simulink model "Control_Seguimiento_de_linea"  (R2023b)
settings: Solver=VariableStepAuto  StartTime=0.0  StopTime=90  RelTol=1e-3
settings Model: Creator=daroc  LastModifiedBy=daroc

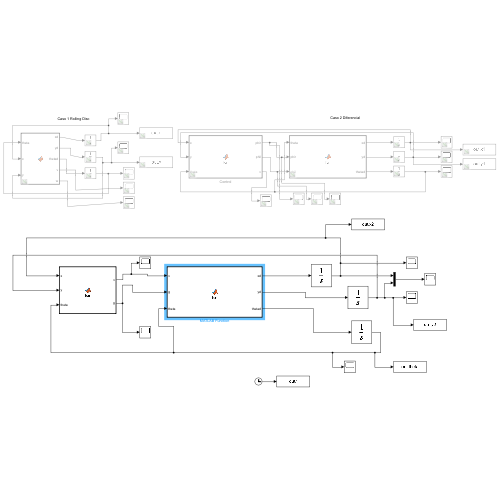
[thumbnail: Simulink's stored preview of the top-level diagram]
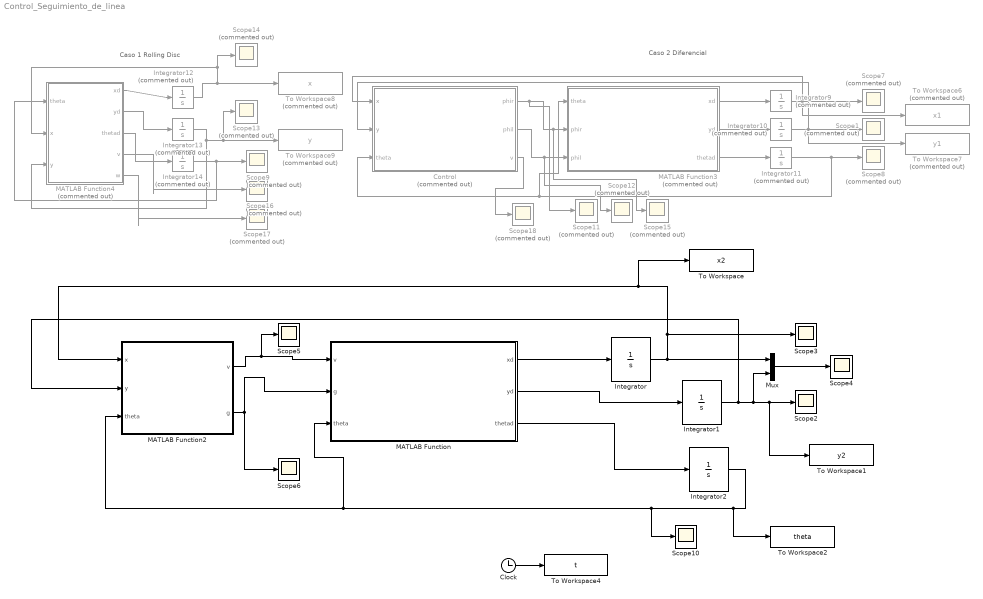
== system Control_Seguimiento_de_linea ==
  note: Caso 1 Rolling Disc
  note: Caso 2 Diferencial
  Clock : Clock
  Control : MATLAB Function  Commented=on  TreatAsAtomicUnit=on
  Integrator : Integrator  InitialCondition=2
  Integrator1 : Integrator  InitialCondition=2
  Integrator{9..14} (6 alike) : Integrator  Commented=on
  Integrator2 : Integrator  InitialCondition=pi/4
  MATLAB Function : MATLAB Function  TreatAsAtomicUnit=on
  MATLAB Function2 : MATLAB Function  TreatAsAtomicUnit=on
  MATLAB Function3 : MATLAB Function  Commented=on  TreatAsAtomicUnit=on
  MATLAB Function4 : MATLAB Function  Commented=on  TreatAsAtomicUnit=on
  Mux : Mux  Inputs=2
  Scope{1,7..9,11..18} (12 alike) : Scope  Commented=on
  Scope{2..6,10} (6 alike) : Scope
  To Workspace : ToWorkspace  VariableName=x2  SampleTime=-1
  To Workspace1 : ToWorkspace  VariableName=y2  SampleTime=-1
  To Workspace2 : ToWorkspace  VariableName=theta  SampleTime=-1
  To Workspace4 : ToWorkspace  VariableName=t  SampleTime=-1
  To Workspace6 : ToWorkspace  Commented=on  VariableName=x1  SampleTime=-1
  To Workspace7 : ToWorkspace  Commented=on  VariableName=y1  SampleTime=-1
  To Workspace8 : ToWorkspace  Commented=on  VariableName=x  SampleTime=-1
  To Workspace9 : ToWorkspace  Commented=on  VariableName=y  SampleTime=-1
  wires:
  MATLAB Function4/1(xd) -> Integrator12/1
  Integrator13/1 -> MATLAB Function4/3(y), Scope13/1, To Workspace9/1
  MATLAB Function4/2(yd) -> Integrator13/1
  Integrator14/1 -> Scope9/1, MATLAB Function4/1(theta)
  Integrator12/1 -> MATLAB Function4/2(x), Scope14/1, To Workspace8/1
  MATLAB Function4/3(thetad) -> Integrator14/1
  Integrator10/1 -> Scope1/1, To Workspace7/1, Control/2(y)
  MATLAB Function3/3(thetad) -> Integrator11/1
  MATLAB Function3/1(xd) -> Integrator9/1
  Integrator11/1 -> MATLAB Function3/1(theta), Control/3(theta), Scope8/1
  Integrator9/1 -> Control/1(x), To Workspace6/1, Scope7/1
  MATLAB Function3/2(yd) -> Integrator10/1
  Control/2(phil) -> Scope12/1, MATLAB Function3/3(phil)
  Control/1(phir) -> Scope11/1, Scope15/1, MATLAB Function3/2(phir)
  MATLAB Function2/1(v) -> MATLAB Function/1(v), Scope5/1
  Integrator2/1 -> To Workspace2/1, Scope10/1, MATLAB Function2/3(theta), MATLAB Function/3(theta)
  Integrator1/1 -> MATLAB Function2/2(y), Mux/2, To Workspace1/1, Scope2/1
  Integrator/1 -> Scope3/1, MATLAB Function2/1(x), To Workspace/1, Mux/1
  MATLAB Function/1(xd) -> Integrator/1
  MATLAB Function/3(thetad) -> Integrator2/1
  MATLAB Function2/2(g) -> Scope6/1, MATLAB Function/2(g)
  Clock/1 -> To Workspace4/1
  Mux/1 -> Scope4/1
  MATLAB Function/2(yd) -> Integrator1/1
  MATLAB Function4/4(v) -> Scope16/1
  MATLAB Function4/5(w) -> Scope17/1
  Control/3(v) -> Scope18/1

== matlab function Control_Seguimiento_de_linea/MATLAB Function ==
  data: v input; xd output; yd output; thetad output; g input; theta input
function [xd,yd,thetad] = fcn(v,g,theta)

L = 0.5;
Rb = L/tan(g);

xd=v*cos(theta);
yd=v*sin(theta);
thetad=v/Rb;

== matlab function Control_Seguimiento_de_linea/Control ==
  data: phir output; phil output; x input; y input; theta input; v output
function [phir,phil,v] = fcn(x,y,theta)

a = 1/5;
b = 1;
c = 1/5;
Kd = 0.7;
Kh = 0.7;
l = 0.5;
r = 0.1;
v = 0.5;

d = ([a b c])*[x; y; 1]/sqrt(a^2+b^2);
alpha_d = -Kd*d;
theta_des = atan2(-a,b);
deltaTheta = theta_des - theta;
alpha_h = Kh*deltaTheta;
w = alpha_d+alpha_h;
phir = (v/r)+(w/r)*(l/2);
phil = (v/r)-(w/r)*(l/2);

== matlab function Control_Seguimiento_de_linea/MATLAB Function2 ==
  data: x input; v output; y input; g output; theta input
function [v, g] = fcn(x,y,theta)

a = 1;
b = 1;
c = -8;
Kd = 0.7;
Kh = 0.7;

v = 0.5;

d = ([a b c])*[x; y; 1]/sqrt(a^2+b^2);
alpha_d = -Kd*d;
theta_des = atan2(-a,b);
deltaTheta = theta_des - theta;
alpha_h = Kh*deltaTheta;

g = alpha_d+alpha_h;

== matlab function Control_Seguimiento_de_linea/MATLAB Function3 ==
  data: xd output; yd output; thetad output; theta input; phir input; phil input
function [xd,yd,thetad] = fcn(theta,phir,phil)

l = 0.5;
r = 0.1;

xd=(r/2)*(phir+phil)*cos(theta);
yd=(r/2)*(phir+phil)*sin(theta);
thetad=(r/l)*(phir-phil);

== matlab function Control_Seguimiento_de_linea/MATLAB Function4 ==
  data: theta input; xd output; yd output; thetad output; x input; y input; v output; w output
function [xd,yd,thetad,v,w] = fcn(theta,x,y)

A=1/5;
B=1;
C=1/5;
k_d=0.7;
k_h=0.7;

d=([A B C])*[x;y;1]/sqrt(A^2+B^2);
alpha_d=-k_d*d;
theta_des=atan2(-A,B);
deltha_theta=theta_des-theta;
alpha_h=k_h*deltha_theta;
v = 0.5;
w = alpha_d+alpha_h;

xd=v*cos(theta);
yd=v*sin(theta);
thetad=w;
